simulink model "DR_01"  (R2022a)
settings: Solver=ode4  StartTime=0.0  StopTime=TMax  FixedStep=DT  MaxStep=DT  RelTol=1e-3  EnableMultiTasking=on
undefined symbols (not defined in the file or in its folder): OutList, strmatch
settings Model: Creator=bjonkman  LastModifiedBy=jgonzalessilva
settings SolverCC: AlgebraicLoopSolver=TrustRegion
settings DataIOCC: SaveFormat=Array  SignalLoggingSaveFormat=ModelDataLogs  SaveOutput=off  SaveTime=off  ReturnWorkspaceOutputs=off  SignalLoggingName=sigsOut
settings OptimizationCC: ExpressionDepthLimit=2147483647  LifeSpan=inf
settings DebuggingCC: SaveWithParameterizedLinksMsg=none  UnderspecifiedInitializationDetection=Classic  MergeDetectMultiDrivingBlocksExec=none  SignalResolutionControl=TryResolveAllWithWarning  MultiTaskDSMMsg=warning  MultiTaskCondExecSysMsg=none  FcnCallInpInsideContextMsg=warning  UnconnectedInputMsg=warning  UnconnectedOutputMsg=warning  UnconnectedLineMsg=warning  StateNameClashWarn=warning  SFUnexpectedBacktrackingDiag=warning  SFNoUnconditionalDefaultTransitionDiag=warning  SFExecutionAtInitializationDiag=none  SFMachineParentedDataDiag=warning  ArithmeticOperatorsInVariantConditions=warning
settings HardwareCC: ProdBitPerPointer=32  ProdBitPerSizeT=32  ProdBitPerPtrDiffT=32  ProdLargestAtomicFloat=None  ProdIntDivRoundTo=Undefined  ProdEndianess=Unspecified  ProdWordSize=32  ProdHWDeviceType=32-bit Generic  TargetUnknown=on
settings ModelReferenceCC: PropagateSignalLabelsOutOfModel=off
settings SFSimCC: SimUseLocalCustomCode=off  CustomCodeUndefinedFunction=UseInterfaceOnly
settings RTWCC: RTWUseLocalCustomCode=off  DLArmComputeVersion=19.05
settings CodeAppCC: StateflowObjectComments=on
settings GRTTargetCC: TargetLangStandard=C89/C90 (ANSI)  ModelReferenceCompliant=off  ParMdlRefBuildCompliant=off  CompOptLevelCompliant=off  ConcurrentExecutionCompliant=off  CombineOutputUpdateFcns=off  MatFileLogging=off  GRTInterface=on
settings ConfigComp: CovMetricSettings=dw  CovSaveCumulativeToWorkspaceVar=on  CovSaveSingleToWorkspaceVar=on  CovExternalEMLEnable=off

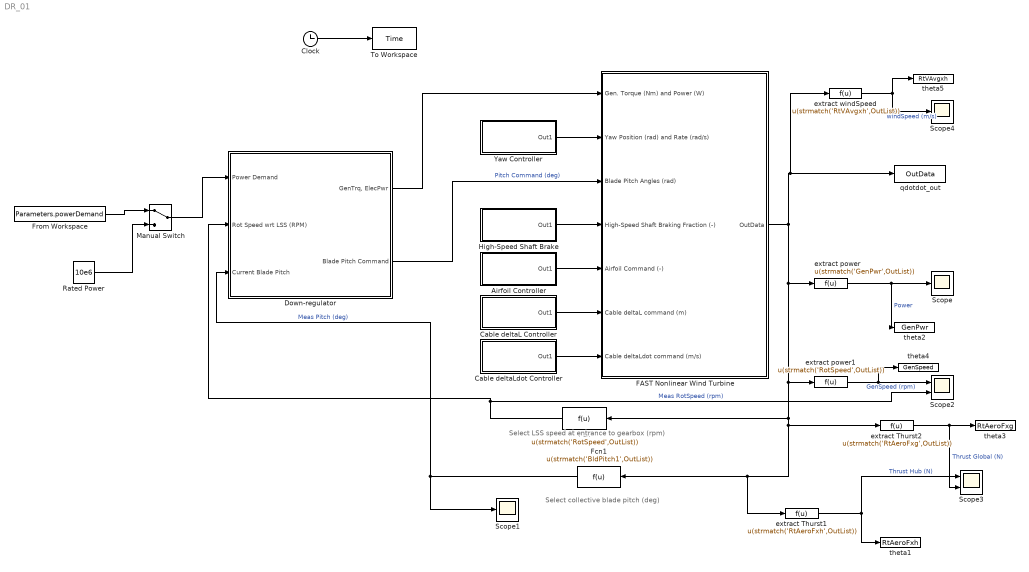
== system DR_01 ==
  note: Select LSS speed at entrance to gearbox (rpm)
  note: Select collective blade pitch (deg)
  Airfoil Controller : Subsystem
  Cable deltaL Controller : Subsystem
  Cable deltaLdot Controller : Subsystem
  Clock : Clock
  Down-regulator : Subsystem
  FAST Nonlinear Wind Turbine : Subsystem  mask(FAST Nonlinear Wind Turbine){}
      mask help: This block contains the FAST S-Function.
      mask init:
      | clear FAST_SFunc
  Fcn : Fcn  Expr=u(strmatch('RotSpeed',OutList))
  Fcn1 : Fcn  Expr=u(strmatch('BldPitch1',OutList))
  From Workspace : FromWorkspace  VariableName=Parameters.powerDemand  SampleTime=-1  Interpolate=off  OutputAfterFinalValue=Holding final value
  High-Speed Shaft Brake : Subsystem
  Manual Switch : ManualSwitch
  Rated Power : Constant  Value=10e6
  Scope : Scope
  Scope1 : Scope
  Scope2 : Scope  NumInputPorts=2
  Scope3 : Scope  NumInputPorts=2
  Scope4 : Scope
  To Workspace : ToWorkspace  VariableName=Time  SampleTime=-1
  Yaw Controller : Subsystem
  extract Thurst1 : Fcn  Expr=u(strmatch('RtAeroFxh',OutList))
  extract Thurst2 : Fcn  Expr=u(strmatch('RtAeroFxg',OutList))
  extract power : Fcn  Expr=u(strmatch('GenPwr',OutList))
  extract power1 : Fcn  Expr=u(strmatch('RotSpeed',OutList))
  extract windSpeed : Fcn  Expr=u(strmatch('RtVAvgxh',OutList))
  qdotdot_out : ToWorkspace  VariableName=OutData  SampleTime=-1
  theta1 : ToWorkspace  VariableName=RtAeroFxh  SampleTime=-1
      settings: MaxDataPoints=Inf
  theta2 : ToWorkspace  VariableName=GenPwr  SampleTime=-1
      settings: MaxDataPoints=Inf
  theta3 : ToWorkspace  VariableName=RtAeroFxg  SampleTime=-1
      settings: MaxDataPoints=Inf
  theta4 : ToWorkspace  VariableName=GenSpeed  SampleTime=-1
      settings: MaxDataPoints=Inf  Decimation=3
  theta5 : ToWorkspace  VariableName=RtVAvgxh  SampleTime=-1
      settings: MaxDataPoints=Inf  Decimation=3
  wires:
  Clock/1 -> To Workspace/1
  Yaw Controller/1(Out1) -> FAST Nonlinear Wind Turbine/2(Yaw Position (rad) and Rate (rad/s))
  High-Speed Shaft Brake/1(Out1) -> FAST Nonlinear Wind Turbine/4(High-Speed Shaft Braking Fraction (-))
  Airfoil Controller/1(Out1) -> FAST Nonlinear Wind Turbine/5(Airfoil Command (-))
  Cable deltaL Controller/1(Out1) -> FAST Nonlinear Wind Turbine/6(Cable deltaL command (m))
  Cable deltaLdot Controller/1(Out1) -> FAST Nonlinear Wind Turbine/7(Cable deltaLdot command (m/s))
  Down-regulator/1("GenTrq, ElecPwr") -> FAST Nonlinear Wind Turbine/1(Gen. Torque (Nm) and Power (W))
  Manual Switch/1 -> Down-regulator/1(Power Demand)
  Rated Power/1 -> Manual Switch/2
  From Workspace/1 -> Manual Switch/1
  Fcn/1 -> Down-regulator/2(Rot Speed wrt LSS (RPM)), Scope2/2  "Meas RotSpeed (rpm)"
  Fcn1/1 -> Down-regulator/3(Current Blade Pitch), Scope1/1  "Meas Pitch (deg)"
  extract power/1 -> theta2/1, Scope/1  "Power"
  extract power1/1 -> theta4/1, Scope2/1  "GenSpeed (rpm)"
  Down-regulator/2(Blade Pitch Command) -> FAST Nonlinear Wind Turbine/3(Blade Pitch Angles (rad))  "Pitch Command (deg)"
  extract Thurst1/1 -> theta1/1, Scope3/1  "Thrust Hub (N)"
  extract windSpeed/1 -> Scope4/1, theta5/1  "windSpeed (m/s)"
  FAST Nonlinear Wind Turbine/1(OutData) -> extract windSpeed/1, qdotdot_out/1, extract power/1, extract power1/1, Fcn/1, extract Thurst2/1, extract Thurst1/1, Fcn1/1
  extract Thurst2/1 -> Scope3/2, theta3/1  "Thrust Global (N)"

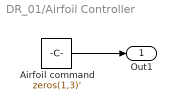
== system DR_01/Airfoil Controller ==
  Airfoil command : Constant  Value=zeros(1,3)'
  Out1 : Outport
  wires:
  Airfoil command/1 -> Out1/1

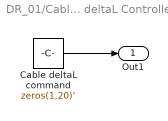
== system DR_01/Cable deltaL Controller ==
  Cable deltaL command : Constant  Value=zeros(1,20)'
  Out1 : Outport
  wires:
  Cable deltaL command/1 -> Out1/1

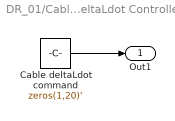
== system DR_01/Cable deltaLdot Controller ==
  Cable deltaLdot command : Constant  Value=zeros(1,20)'
  Out1 : Outport
  wires:
  Cable deltaLdot command/1 -> Out1/1

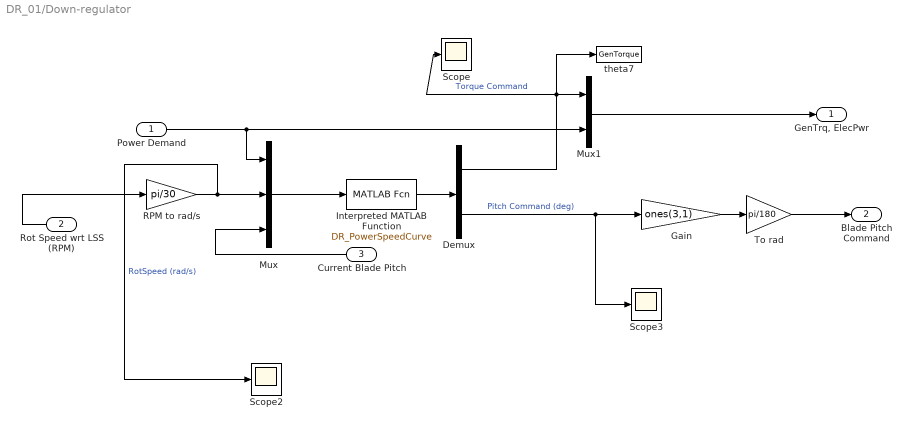
== system DR_01/Down-regulator ==
  Power Demand : Inport
  Rot Speed wrt LSS (RPM) : Inport  Port=2
  Current Blade Pitch : Inport  Port=3
  Demux : Demux  Outputs=2
  Gain : Gain  Gain=ones(3,1)
  Interpreted MATLAB Function : MATLABFcn  MATLABFcn=DR_PowerSpeedCurve  OutputDimensions=2
  Mux : Mux  Inputs=3
  Mux1 : Mux  Inputs=2
  RPM to rad/s : Gain  Gain=pi/30  SaturateOnIntegerOverflow=on  OutDataTypeStr=Inherit: Same as input  ParamDataTypeStr=Inherit: Same as input
  Scope : Scope
  Scope2 : Scope
  Scope3 : Scope
  To rad : Gain  Gain=pi/180
  theta7 : ToWorkspace  VariableName=GenTorque  SampleTime=-1
      settings: MaxDataPoints=Inf
  "GenTrq, ElecPwr" : Outport
  Blade Pitch Command : Outport  Port=2
  wires:
  RPM to rad/s/1 -> Scope2/1, Mux/2  "RotSpeed (rad/s)"
  Mux1/1 -> "GenTrq, ElecPwr"/1
  Interpreted MATLAB Function/1 -> Demux/1
  Current Blade Pitch/1 -> Mux/3
  Mux/1 -> Interpreted MATLAB Function/1
  Power Demand/1 -> Mux1/2, Mux/1
  Demux/1 -> theta7/1, Mux1/1, Scope/1  "Torque Command"
  To rad/1 -> Blade Pitch Command/1
  Gain/1 -> To rad/1
  Demux/2 -> Scope3/1, Gain/1  "Pitch Command (deg)"
  Rot Speed wrt LSS (RPM)/1 -> RPM to rad/s/1

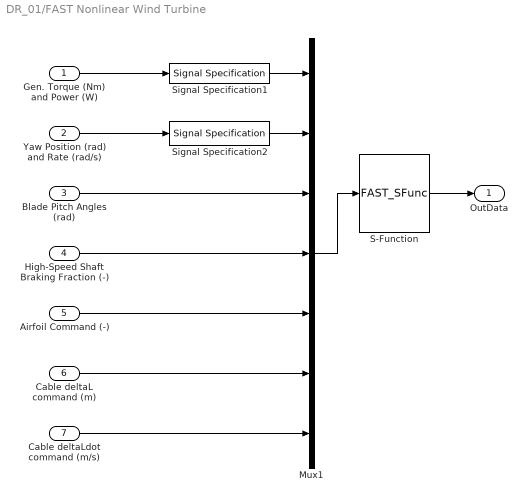
== system DR_01/FAST Nonlinear Wind Turbine ==
  Gen. Torque (Nm) and Power (W) : Inport
  Yaw Position (rad) and Rate (rad/s) : Inport  Port=2
  Blade Pitch Angles (rad) : Inport  Port=3
  High-Speed Shaft Braking Fraction (-) : Inport  Port=4
  Airfoil Command (-) : Inport  Port=5
  Cable deltaL command (m) : Inport  Port=6
  Cable deltaLdot command (m/s) : Inport  Port=7
  Mux1 : Mux  Inputs=7
  S-Function : S-Function  FunctionName=FAST_SFunc  Parameters=FAST_InputFileName, TMax, 0  SFunctionDeploymentMode=off  EnableBusSupport=off
  Signal Specification1 : SignalSpecification  OutDataTypeStr=double  Dimensions=2
  Signal Specification2 : SignalSpecification  OutDataTypeStr=double  Dimensions=2
  OutData : Outport
  wires:
  Gen. Torque (Nm) and Power (W)/1 -> Signal Specification1/1
  S-Function/1 -> OutData/1
  Mux1/1 -> S-Function/1
  Blade Pitch Angles (rad)/1 -> Mux1/3
  Yaw Position (rad) and Rate (rad/s)/1 -> Signal Specification2/1
  Signal Specification1/1 -> Mux1/1
  Signal Specification2/1 -> Mux1/2
  High-Speed Shaft Braking Fraction (-)/1 -> Mux1/4
  Airfoil Command (-)/1 -> Mux1/5
  Cable deltaL command (m)/1 -> Mux1/6
  Cable deltaLdot command (m/s)/1 -> Mux1/7

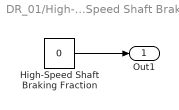
== system DR_01/High-Speed Shaft Brake ==
  High-Speed Shaft Braking Fraction : Constant  Value=0
  Out1 : Outport
  wires:
  High-Speed Shaft Braking Fraction/1 -> Out1/1

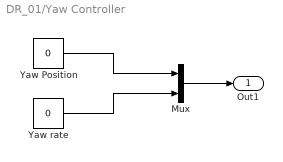
== system DR_01/Yaw Controller ==
  Mux : Mux  Inputs=2
  Yaw Position : Constant  Value=0
  Yaw rate : Constant  Value=0
  Out1 : Outport
  wires:
  Mux/1 -> Out1/1
  Yaw Position/1 -> Mux/1
  Yaw rate/1 -> Mux/2
